simulink model "satellite"  (R2017a)
settings: Solver=FixedStepDiscrete  StartTime=0.0  StopTime=0.02  RelTol=1e-3
libraries: dspswit3 x9, commsynccomp2 x6, dspindex x3, commutil2 x3, dspmathops x3
(part 2 of 15)

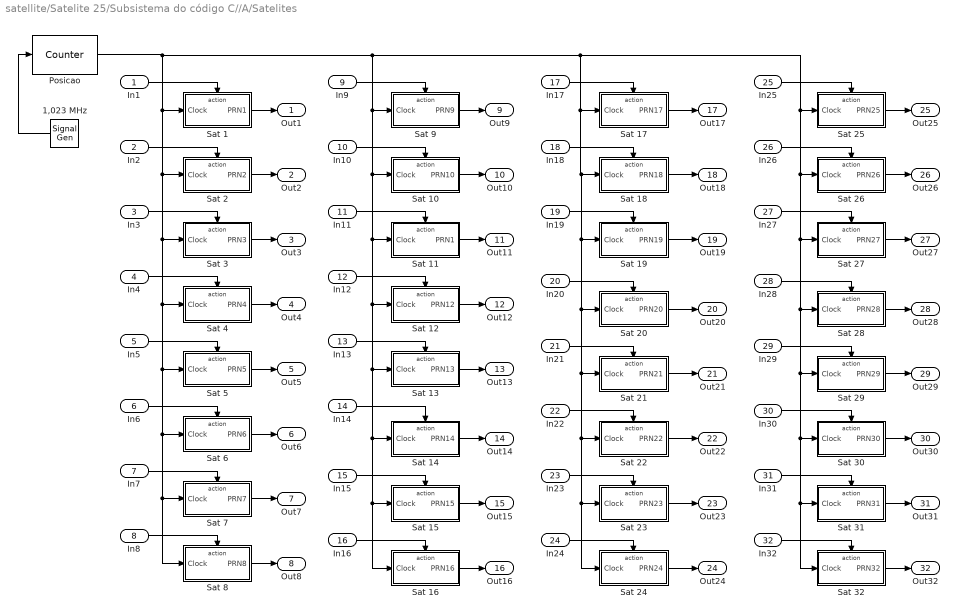
== system satellite/Satelite 25/Subsistema do código C//A/Satelites ==
  In1 : Inport
  In2 : Inport  Port=2
  In3 : Inport  Port=3
  In4 : Inport  Port=4
  In5 : Inport  Port=5
  In6 : Inport  Port=6
  In7 : Inport  Port=7
  In8 : Inport  Port=8
  In9 : Inport  Port=9
  In10 : Inport  Port=10
  In11 : Inport  Port=11
  In12 : Inport  Port=12
  In13 : Inport  Port=13
  In14 : Inport  Port=14
  In15 : Inport  Port=15
  In16 : Inport  Port=16
  In17 : Inport  Port=17
  In18 : Inport  Port=18
  In19 : Inport  Port=19
  In20 : Inport  Port=20
  In21 : Inport  Port=21
  In22 : Inport  Port=22
  In23 : Inport  Port=23
  In24 : Inport  Port=24
  In25 : Inport  Port=25
  In26 : Inport  Port=26
  In27 : Inport  Port=27
  In28 : Inport  Port=28
  In29 : Inport  Port=29
  In30 : Inport  Port=30
  In31 : Inport  Port=31
  In32 : Inport  Port=32
  1,023 MHz : SignalGenerator  WaveForm=square  Frequency=1.023e6
  Posicao : dspswit3/Counter  Direction=Up  CountEvent=Rising edge  CounterSize=User defined  MaxCount=1022  InitialCount=0  Output=Count  HitValue=32  ResetInput=off  SamplesPerFrame=1  Ts=1  CntDtype=double  HitDtype=Logical
  Sat 1 : Subsystem  TreatAsAtomicUnit=on
  Sat 10 : Subsystem  TreatAsAtomicUnit=on
  Sat 11 : Subsystem  TreatAsAtomicUnit=on
  Sat 12 : Subsystem  TreatAsAtomicUnit=on
  Sat 13 : Subsystem  TreatAsAtomicUnit=on
  Sat 14 : Subsystem  TreatAsAtomicUnit=on
  Sat 15 : Subsystem  TreatAsAtomicUnit=on
  Sat 16 : Subsystem  TreatAsAtomicUnit=on
  Sat 17 : Subsystem  TreatAsAtomicUnit=on
  Sat 18 : Subsystem  TreatAsAtomicUnit=on
  Sat 19 : Subsystem  TreatAsAtomicUnit=on
  Sat 2 : Subsystem  TreatAsAtomicUnit=on
  Sat 20 : Subsystem  TreatAsAtomicUnit=on
  Sat 21 : Subsystem  TreatAsAtomicUnit=on
  Sat 22 : Subsystem  TreatAsAtomicUnit=on
  Sat 23 : Subsystem  TreatAsAtomicUnit=on
  Sat 24 : Subsystem  TreatAsAtomicUnit=on
  Sat 25 : Subsystem  TreatAsAtomicUnit=on
  Sat 26 : Subsystem  TreatAsAtomicUnit=on
  Sat 27 : Subsystem  TreatAsAtomicUnit=on
  Sat 28 : Subsystem  TreatAsAtomicUnit=on
  Sat 29 : Subsystem  TreatAsAtomicUnit=on
  Sat 3 : Subsystem  TreatAsAtomicUnit=on
  Sat 30 : Subsystem  TreatAsAtomicUnit=on
  Sat 31 : Subsystem  TreatAsAtomicUnit=on
  Sat 32 : Subsystem  TreatAsAtomicUnit=on
  Sat 4 : Subsystem  TreatAsAtomicUnit=on
  Sat 5 : Subsystem  TreatAsAtomicUnit=on
  Sat 6 : Subsystem  TreatAsAtomicUnit=on
  Sat 7 : Subsystem  TreatAsAtomicUnit=on
  Sat 8 : Subsystem  TreatAsAtomicUnit=on
  Sat 9 : Subsystem  TreatAsAtomicUnit=on
  Out1 : Outport
  Out2 : Outport  Port=2
  Out3 : Outport  Port=3
  Out4 : Outport  Port=4
  Out5 : Outport  Port=5
  Out6 : Outport  Port=6
  Out7 : Outport  Port=7
  Out8 : Outport  Port=8
  Out9 : Outport  Port=9
  Out10 : Outport  Port=10
  Out11 : Outport  Port=11
  Out12 : Outport  Port=12
  Out13 : Outport  Port=13
  Out14 : Outport  Port=14
  Out15 : Outport  Port=15
  Out16 : Outport  Port=16
  Out17 : Outport  Port=17
  Out18 : Outport  Port=18
  Out19 : Outport  Port=19
  Out20 : Outport  Port=20
  Out21 : Outport  Port=21
  Out22 : Outport  Port=22
  Out23 : Outport  Port=23
  Out24 : Outport  Port=24
  Out25 : Outport  Port=25
  Out26 : Outport  Port=26
  Out27 : Outport  Port=27
  Out28 : Outport  Port=28
  Out29 : Outport  Port=29
  Out30 : Outport  Port=30
  Out31 : Outport  Port=31
  Out32 : Outport  Port=32
  wires:
  Sat 1/1(PRN1) -> Out1/1
  Sat 2/1(PRN2) -> Out2/1
  Sat 3/1(PRN3) -> Out3/1
  Sat 4/1(PRN4) -> Out4/1
  Sat 5/1(PRN5) -> Out5/1
  Sat 6/1(PRN6) -> Out6/1
  In1/1 -> Sat 1/Action
  In2/1 -> Sat 2/Action
  In3/1 -> Sat 3/Action
  In4/1 -> Sat 4/Action
  In5/1 -> Sat 5/Action
  In6/1 -> Sat 6/Action
  In8/1 -> Sat 8/Action
  In10/1 -> Sat 10/Action
  In7/1 -> Sat 7/Action
  Sat 8/1(PRN8) -> Out8/1
  Sat 11/1(PRN1) -> Out11/1
  Sat 10/1(PRN10) -> Out10/1
  In11/1 -> Sat 11/Action
  In9/1 -> Sat 9/Action
  Sat 12/1(PRN12) -> Out12/1
  Sat 9/1(PRN9) -> Out9/1
  Sat 7/1(PRN7) -> Out7/1
  In12/1 -> Sat 12/Action
  In14/1 -> Sat 14/Action
  In16/1 -> Sat 16/Action
  In13/1 -> Sat 13/Action
  Sat 14/1(PRN14) -> Out14/1
  Sat 17/1(PRN17) -> Out17/1
  Sat 16/1(PRN16) -> Out16/1
  In17/1 -> Sat 17/Action
  In15/1 -> Sat 15/Action
  Sat 18/1(PRN18) -> Out18/1
  Sat 15/1(PRN15) -> Out15/1
  Sat 13/1(PRN13) -> Out13/1
  In18/1 -> Sat 18/Action
  In20/1 -> Sat 20/Action
  In22/1 -> Sat 22/Action
  In19/1 -> Sat 19/Action
  Sat 20/1(PRN20) -> Out20/1
  Sat 23/1(PRN23) -> Out23/1
  Sat 22/1(PRN22) -> Out22/1
  In23/1 -> Sat 23/Action
  In21/1 -> Sat 21/Action
  Sat 24/1(PRN24) -> Out24/1
  Sat 21/1(PRN21) -> Out21/1
  Sat 19/1(PRN19) -> Out19/1
  In24/1 -> Sat 24/Action
  In26/1 -> Sat 26/Action
  In28/1 -> Sat 28/Action
  In25/1 -> Sat 25/Action
  Sat 26/1(PRN26) -> Out26/1
  Sat 29/1(PRN29) -> Out29/1
  Sat 28/1(PRN28) -> Out28/1
  In29/1 -> Sat 29/Action
  In27/1 -> Sat 27/Action
  Sat 30/1(PRN30) -> Out30/1
  Sat 27/1(PRN27) -> Out27/1
  Sat 25/1(PRN25) -> Out25/1
  In30/1 -> Sat 30/Action
  In32/1 -> Sat 32/Action
  Sat 32/1(PRN32) -> Out32/1
  Sat 31/1(PRN31) -> Out31/1
  In31/1 -> Sat 31/Action
  Posicao/1 -> Sat 8/1(Clock), Sat 7/1(Clock), Sat 6/1(Clock), Sat 5/1(Clock), Sat 4/1(Clock), Sat 3/1(Clock), Sat 2/1(Clock), Sat 1/1(Clock), Sat 25/1(Clock), Sat 26/1(Clock), Sat 28/1(Clock), Sat 29/1(Clock), Sat 30/1(Clock), Sat 31/1(Clock), Sat 32/1(Clock), Sat 27/1(Clock), Sat 24/1(Clock), Sat 23/1(Clock), Sat 22/1(Clock), Sat 21/1(Clock), Sat 20/1(Clock), Sat 19/1(Clock), Sat 18/1(Clock), Sat 17/1(Clock), Sat 9/1(Clock), Sat 10/1(Clock), Sat 16/1(Clock), Sat 15/1(Clock), Sat 14/1(Clock), Sat 13/1(Clock), Sat 12/1(Clock), Sat 11/1(Clock)
  1,023 MHz/1 -> Posicao/1

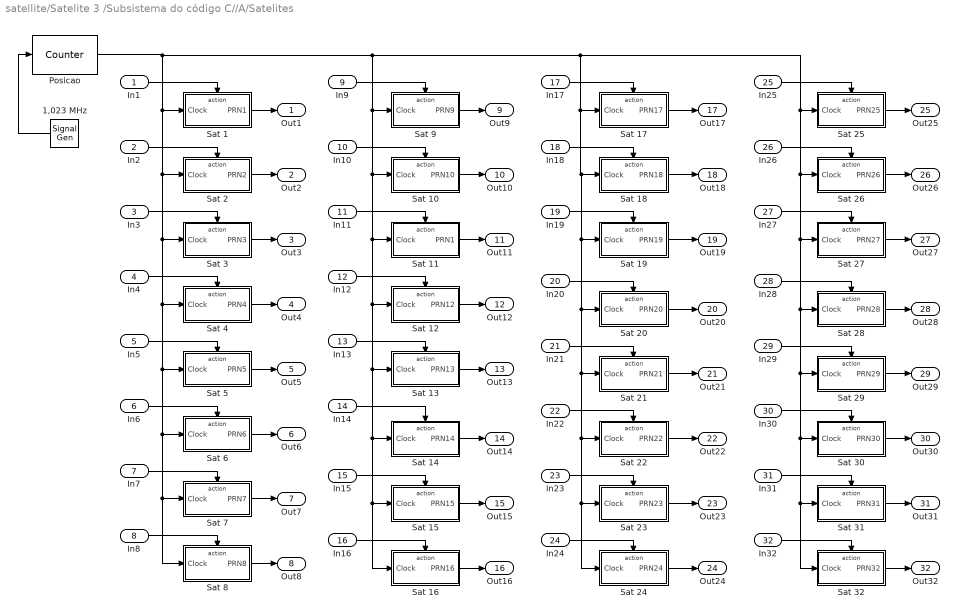
== system satellite/Satelite 3 /Subsistema do código C//A/Satelites ==
  In1 : Inport
  In2 : Inport  Port=2
  In3 : Inport  Port=3
  In4 : Inport  Port=4
  In5 : Inport  Port=5
  In6 : Inport  Port=6
  In7 : Inport  Port=7
  In8 : Inport  Port=8
  In9 : Inport  Port=9
  In10 : Inport  Port=10
  In11 : Inport  Port=11
  In12 : Inport  Port=12
  In13 : Inport  Port=13
  In14 : Inport  Port=14
  In15 : Inport  Port=15
  In16 : Inport  Port=16
  In17 : Inport  Port=17
  In18 : Inport  Port=18
  In19 : Inport  Port=19
  In20 : Inport  Port=20
  In21 : Inport  Port=21
  In22 : Inport  Port=22
  In23 : Inport  Port=23
  In24 : Inport  Port=24
  In25 : Inport  Port=25
  In26 : Inport  Port=26
  In27 : Inport  Port=27
  In28 : Inport  Port=28
  In29 : Inport  Port=29
  In30 : Inport  Port=30
  In31 : Inport  Port=31
  In32 : Inport  Port=32
  1,023 MHz : SignalGenerator  WaveForm=square  Frequency=1.023e6
  Posicao : dspswit3/Counter  Direction=Up  CountEvent=Rising edge  CounterSize=User defined  MaxCount=1022  InitialCount=0  Output=Count  HitValue=32  ResetInput=off  SamplesPerFrame=1  Ts=1  CntDtype=double  HitDtype=Logical
  Sat 1 : Subsystem  TreatAsAtomicUnit=on
  Sat 10 : Subsystem  TreatAsAtomicUnit=on
  Sat 11 : Subsystem  TreatAsAtomicUnit=on
  Sat 12 : Subsystem  TreatAsAtomicUnit=on
  Sat 13 : Subsystem  TreatAsAtomicUnit=on
  Sat 14 : Subsystem  TreatAsAtomicUnit=on
  Sat 15 : Subsystem  TreatAsAtomicUnit=on
  Sat 16 : Subsystem  TreatAsAtomicUnit=on
  Sat 17 : Subsystem  TreatAsAtomicUnit=on
  Sat 18 : Subsystem  TreatAsAtomicUnit=on
  Sat 19 : Subsystem  TreatAsAtomicUnit=on
  Sat 2 : Subsystem  TreatAsAtomicUnit=on
  Sat 20 : Subsystem  TreatAsAtomicUnit=on
  Sat 21 : Subsystem  TreatAsAtomicUnit=on
  Sat 22 : Subsystem  TreatAsAtomicUnit=on
  Sat 23 : Subsystem  TreatAsAtomicUnit=on
  Sat 24 : Subsystem  TreatAsAtomicUnit=on
  Sat 25 : Subsystem  TreatAsAtomicUnit=on
  Sat 26 : Subsystem  TreatAsAtomicUnit=on
  Sat 27 : Subsystem  TreatAsAtomicUnit=on
  Sat 28 : Subsystem  TreatAsAtomicUnit=on
  Sat 29 : Subsystem  TreatAsAtomicUnit=on
  Sat 3 : Subsystem  TreatAsAtomicUnit=on
  Sat 30 : Subsystem  TreatAsAtomicUnit=on
  Sat 31 : Subsystem  TreatAsAtomicUnit=on
  Sat 32 : Subsystem  TreatAsAtomicUnit=on
  Sat 4 : Subsystem  TreatAsAtomicUnit=on
  Sat 5 : Subsystem  TreatAsAtomicUnit=on
  Sat 6 : Subsystem  TreatAsAtomicUnit=on
  Sat 7 : Subsystem  TreatAsAtomicUnit=on
  Sat 8 : Subsystem  TreatAsAtomicUnit=on
  Sat 9 : Subsystem  TreatAsAtomicUnit=on
  Out1 : Outport
  Out2 : Outport  Port=2
  Out3 : Outport  Port=3
  Out4 : Outport  Port=4
  Out5 : Outport  Port=5
  Out6 : Outport  Port=6
  Out7 : Outport  Port=7
  Out8 : Outport  Port=8
  Out9 : Outport  Port=9
  Out10 : Outport  Port=10
  Out11 : Outport  Port=11
  Out12 : Outport  Port=12
  Out13 : Outport  Port=13
  Out14 : Outport  Port=14
  Out15 : Outport  Port=15
  Out16 : Outport  Port=16
  Out17 : Outport  Port=17
  Out18 : Outport  Port=18
  Out19 : Outport  Port=19
  Out20 : Outport  Port=20
  Out21 : Outport  Port=21
  Out22 : Outport  Port=22
  Out23 : Outport  Port=23
  Out24 : Outport  Port=24
  Out25 : Outport  Port=25
  Out26 : Outport  Port=26
  Out27 : Outport  Port=27
  Out28 : Outport  Port=28
  Out29 : Outport  Port=29
  Out30 : Outport  Port=30
  Out31 : Outport  Port=31
  Out32 : Outport  Port=32
  wires:
  Sat 1/1(PRN1) -> Out1/1
  Sat 2/1(PRN2) -> Out2/1
  Sat 3/1(PRN3) -> Out3/1
  Sat 4/1(PRN4) -> Out4/1
  Sat 5/1(PRN5) -> Out5/1
  Sat 6/1(PRN6) -> Out6/1
  In1/1 -> Sat 1/Action
  In2/1 -> Sat 2/Action
  In3/1 -> Sat 3/Action
  In4/1 -> Sat 4/Action
  In5/1 -> Sat 5/Action
  In6/1 -> Sat 6/Action
  In8/1 -> Sat 8/Action
  In10/1 -> Sat 10/Action
  In7/1 -> Sat 7/Action
  Sat 8/1(PRN8) -> Out8/1
  Sat 11/1(PRN1) -> Out11/1
  Sat 10/1(PRN10) -> Out10/1
  In11/1 -> Sat 11/Action
  In9/1 -> Sat 9/Action
  Sat 12/1(PRN12) -> Out12/1
  Sat 9/1(PRN9) -> Out9/1
  Sat 7/1(PRN7) -> Out7/1
  In12/1 -> Sat 12/Action
  In14/1 -> Sat 14/Action
  In16/1 -> Sat 16/Action
  In13/1 -> Sat 13/Action
  Sat 14/1(PRN14) -> Out14/1
  Sat 17/1(PRN17) -> Out17/1
  Sat 16/1(PRN16) -> Out16/1
  In17/1 -> Sat 17/Action
  In15/1 -> Sat 15/Action
  Sat 18/1(PRN18) -> Out18/1
  Sat 15/1(PRN15) -> Out15/1
  Sat 13/1(PRN13) -> Out13/1
  In18/1 -> Sat 18/Action
  In20/1 -> Sat 20/Action
  In22/1 -> Sat 22/Action
  In19/1 -> Sat 19/Action
  Sat 20/1(PRN20) -> Out20/1
  Sat 23/1(PRN23) -> Out23/1
  Sat 22/1(PRN22) -> Out22/1
  In23/1 -> Sat 23/Action
  In21/1 -> Sat 21/Action
  Sat 24/1(PRN24) -> Out24/1
  Sat 21/1(PRN21) -> Out21/1
  Sat 19/1(PRN19) -> Out19/1
  In24/1 -> Sat 24/Action
  In26/1 -> Sat 26/Action
  In28/1 -> Sat 28/Action
  In25/1 -> Sat 25/Action
  Sat 26/1(PRN26) -> Out26/1
  Sat 29/1(PRN29) -> Out29/1
  Sat 28/1(PRN28) -> Out28/1
  In29/1 -> Sat 29/Action
  In27/1 -> Sat 27/Action
  Sat 30/1(PRN30) -> Out30/1
  Sat 27/1(PRN27) -> Out27/1
  Sat 25/1(PRN25) -> Out25/1
  In30/1 -> Sat 30/Action
  In32/1 -> Sat 32/Action
  Sat 32/1(PRN32) -> Out32/1
  Sat 31/1(PRN31) -> Out31/1
  In31/1 -> Sat 31/Action
  Posicao/1 -> Sat 8/1(Clock), Sat 7/1(Clock), Sat 6/1(Clock), Sat 5/1(Clock), Sat 4/1(Clock), Sat 3/1(Clock), Sat 2/1(Clock), Sat 1/1(Clock), Sat 25/1(Clock), Sat 26/1(Clock), Sat 28/1(Clock), Sat 29/1(Clock), Sat 30/1(Clock), Sat 31/1(Clock), Sat 32/1(Clock), Sat 27/1(Clock), Sat 24/1(Clock), Sat 23/1(Clock), Sat 22/1(Clock), Sat 21/1(Clock), Sat 20/1(Clock), Sat 19/1(Clock), Sat 18/1(Clock), Sat 17/1(Clock), Sat 9/1(Clock), Sat 10/1(Clock), Sat 16/1(Clock), Sat 15/1(Clock), Sat 14/1(Clock), Sat 13/1(Clock), Sat 12/1(Clock), Sat 11/1(Clock)
  1,023 MHz/1 -> Posicao/1

== system satellite/Satelite 14 /Subsistema do código C//A/Satelites/Sat 1 ==
  Clock : Inport
  Action Port : ActionPort  ActionType=case
  Tabela de C/A : Lookup_n-D  NumberOfTableDimensions=1  BreakpointsForDimension1=[0,1,2,3,4,5,6,7,8,9,10,11,12,13,14,15,16,17,18,19,20,21,22,23,24,25,26,27,28,29,30,31,32,33,34,35,36,37,38,39,40,41,42,43,44,45,46,47,48,49,50,51,52,53,54,55,56,57,58,59,60,61,62,63,64,65,66,67,68,69,70,71,72,73,74,75,76,77,78,79,80,81,82,83,84,85,86,87,88,89,90,91,92,93,94,95,96,97,98,99,100,101,102,103,104,105,106,107,108,109,110,111,112,113,114,115,116,117,118,119,120,121,122,123,124,125,126,127,128,129,130,131,132,133,134,135,136,137,138,139,140,141,142,143,144,145,146,147,148,149,150,151,152,153,154,155,156,157,158,159,160,161,162,163,164,165,166,167,168,169,170,171,172,173,174,175,176,177,178,179,180,181,182,183,184,185,186,187,188,189,190,191,192,193,194,195,196,197,198,199,200,201,202,203,204,205,206,207,208,209,210,211,212,213,214,215,216,217,218,219,220,221,222,223,224,225,226,227,228,229,230,231,232,233,234,235,236,237,238,239,240,241,242,243,244,245,246,247,248,249,250,251,252,253,254,255,256,257,258,259,260,261,262,263,264,265,266,267,268,269,270,271,272,273,274,275,276,277,278,279,280,281,282,283,284,285,286,287,288,289,290,291,292,293,294,295,296,297,298,299,300,301,302,303,304,305,306,307,308,309,310,311,312,313,314,315,316,317,318,319,320,321,322,323,324,325,326,327,328,329,330,331,332,333,334,335,336,337,338,339,340,341,342,343,344,345,346,347,348,349,350,351,352,353,354,355,356,357,358,359,360,361,362,363,364,365,366,367,368,369,370,371,372,373,374,375,376,377,378,379,380,381,382,383,384,385,386,387,388,389,390,391,392,393,394,395,396,397,398,399,400,401,402,403,404,405,406,407,408,409,410,411,412,413,414,415,416,417,418,419,420,421,422,423,424,425,426,427,428,429,430,431,432,433,434,435,436,437,438,439,440,441,442,443,444,445,446,447,448,449,450,451,452,453,454,455,456,457,458,459,460,461,462,463,464,465,466,467,468,469,470,471,472,473,474,475,476,477,478,479,480,481,482,483,484,485,486,487,488,489,490,491,492,493,494,495,496,497,498,499,500,501,502,503,504,505,506,507,508,509,510,511,512,513,514,515,516,517,518,519,520,521,522,523,524,525,526,527,528,529,530,531,532,533,534,535,536,537,538,539,540,541,542,543,544,545,546,547,548,549,550,551,552,553,554,555,556,557,558,559,560,561,562,563,564,565,566,567,568,569,570,571,572,573,574,575,576,577,578,579,580,581,582,583,584,585,586,587,588,589,590,591,592,593,594,595,596,597,598,599,600,601,602,603,604,605,606,607,608,609,610,611,612,613,614,615,616,617,618,619,620,621,622,623,624,625,626,627,628,629,630,631,632,633,634,635,636,637,638,639,640,641,642,643,644,645,646,647,648,649,650,651,652,653,654,655,656,657,658,659,660,661,662,663,664,665,666,667,668,669,670,671,672,673,674,675,676,677,678,679,680,681,682,683,684,685,686,687,688,689,690,691,692,693,694,695,696,697,698,699,700,701,702,703,704,705,706,707,708,709,710,711,712,713,714,715,716,717,718,719,720,721,722,723,724,725,726,727,728,729,730,731,732,733,734,735,736,737,738,739,740,741,742,743,744,745,746,747,748,749,750,751,752,753,754,755,756,757,758,759,760,761,762,763,764,765,766,767,768,769,770,771,772,773,774,775,776,777,778,779,780,781,782,783,784,785,786,787,788,789,790,791,792,793,794,795,796,797,798,799,800,801,802,803,804,805,806,807,808,809,810,811,812,813,814,815,816,817,818,819,820,821,822,823,824,825,826,827,828,829,830,831,832,833,834,835,836,837,838,839,840,841,842,843,844,845,846,847,848,849,850,851,852,853,854,855,856,857,858,859,860,861,862,863,864,865,866,867,868,869,870,871,872,873,874,875,876,877,878,879,880,881,882,883,884,885,886,887,888,889,890,891,892,893,894,895,896,897,898,899,900,901,902,903,904,905,906,907,908,909,910,911,912,913,914,915,916,917,918,919,920,921,922,923,924,925,926,927,928,929,930,931,932,933,934,935,936,937,938,939,940,941,942,943,944,945,946,947,948,949,950,951,952,953,954,955,956,957,958,959,960,961,962,963,964,965,966,967,968,969,970,971,972,973,974,975,976,977,978,979,980,981,982,983,984,985,986,987,988,989,990,991,992,993,994,995,996,997,998,999,1000,1001,1002,1003,1004,1005,1006,1007,1008,1009,1010,1011,1012,1013,1014,1015,1016,1017,1018,1019,1020,1021,1022]  Table=[1,1,-1,-1,1,-1,-1,-1,-1,-1,1,1,1,-1,-1,1,-1,1,-1,-1,1,-1,-1,1,1,1,1,-1,-1,1,-1,1,-1,-1,-1,1,-1,-1,1,1,1,1,1,-1,1,-1,1,-1,1,1,-1,1,-1,-1,-1,1,-1,-1,-1,1,-1,1,-1,1,-1,1,-1,1,1,-1,-1,1,-1,-1,-1,1,1,1,1,-1,1,-1,-1,1,1,1,1,1,1,-1,1,1,-1,1,1,1,-1,-1,1,1,-1,1,1,1,1,1,-1,-1,1,-1,1,-1,1,-1,1,-1,-1,-1,-1,1,-1,-1,-1,-1,-1,-1,-1,-1,1,1,1,-1,1,-1,1,-1,-1,1,-1,-1,-1,1,-1,-1,1,1,-1,1,1,1,1,-1,-1,-1,-1,-1,1,1,1,1,-1,1,-1,1,1,1,-1,-1,1,1,-1,-1,1,1,1,1,-1,1,1,-1,-1,-1,-1,-1,-1,-1,1,-1,1,1,1,1,-1,-1,1,1,1,1,1,-1,1,-1,1,-1,-1,1,1,-1,-1,-1,1,-1,1,1,-1,1,1,1,-1,-1,-1,1,1,-1,1,1,1,1,-1,1,-1,1,-1,-1,-1,1,-1,1,-1,1,1,-1,-1,-1,-1,-1,1,-1,-1,-1,-1,-1,-1,-1,-1,1,-1,-1,-1,-1,-1,-1,1,1,-1,-1,-1,1,1,1,-1,1,1,-1,-1,-1,-1,-1,-1,1,1,1,-1,-1,-1,1,1,-1,1,1,1,1,1,1,1,1,1,-1,1,-1,-1,1,1,1,-1,1,-1,-1,1,-1,1,1,-1,1,1,-1,-1,-1,-1,1,-1,1,-1,1,-1,1,1,-1,-1,-1,1,-1,-1,1,1,1,-1,-1,1,-1,1,1,-1,1,1,1,-1,1,1,-1,-1,-1,1,1,1,-1,1,1,1,-1,1,1,1,1,-1,-1,-1,-1,1,1,-1,1,1,-1,-1,-1,-1,1,1,-1,-1,1,-1,-1,1,-1,-1,1,-1,-1,-1,-1,-1,1,1,-1,1,1,-1,1,-1,-1,1,-1,1,1,-1,1,1,1,1,-1,-1,-1,1,-1,1,1,1,-1,-1,-1,-1,-1,-1,1,-1,1,-1,-1,1,-1,-1,1,1,1,1,1,1,-1,-1,-1,-1,-1,1,-1,1,-1,1,-1,1,1,1,-1,-1,1,1,1,1,1,-1,1,-1,1,1,1,1,1,-1,-1,1,1,-1,-1,1,1,-1,-1,-1,1,1,1,-1,-1,-1,1,1,-1,1,1,-1,1,-1,1,-1,1,-1,1,1,-1,1,1,-1,-1,-1,1,1,-1,1,1,1,-1,1,1,1,-1,-1,-1,-1,-1,-1,-1,-1,-1,-1,-1,1,-1,1,1,-1,-1,1,1,-1,1,1,-1,-1,1,1,1,-1,1,1,-1,1,-1,-1,-1,-1,-1,1,-1,1,-1,1,-1,1,1,1,-1,1,-1,1,1,1,-1,1,-1,-1,1,-1,1,-1,-1,-1,1,1,1,-1,-1,1,1,1,-1,-1,-1,1,-1,-1,1,-1,1,-1,-1,-1,1,-1,1,-1,-1,1,-1,1,1,-1,1,-1,-1,-1,-1,1,-1,1,-1,1,1,-1,1,1,-1,1,-1,1,1,-1,1,1,-1,-1,-1,1,1,1,-1,-1,1,1,1,1,-1,1,1,-1,-1,1,-1,-1,-1,-1,1,1,1,1,1,1,-1,-1,1,-1,1,1,-1,1,-1,-1,-1,1,-1,-1,-1,-1,1,1,1,1,1,-1,1,-1,1,-1,1,1,1,-1,-1,1,1,-1,-1,1,-1,-1,1,-1,-1,1,-1,-1,1,-1,1,1,1,1,1,1,1,1,1,1,-1,-1,-1,-1,1,1,1,1,1,-1,1,1,1,1,-1,-1,-1,1,1,-1,1,1,1,-1,-1,1,-1,1,1,-1,-1,-1,-1,1,1,1,-1,-1,1,-1,1,-1,1,-1,-1,-1,-1,1,-1,1,-1,-1,1,-1,1,-1,1,1,1,1,1,1,-1,-1,-1,1,1,1,1,-1,1,1,-1,1,-1,-1,1,1,1,-1,1,1,-1,-1,1,1,1,1,1,1,-1,1,1,1,1,1,-1,1,-1,-1,-1,1,1,-1,-1,-1,1,1,1,1,1,-1,-1,-1,-1,-1,-1,-1,1,-1,-1,1,-1,1,-1,-1,-1,1,-1,1,1,-1,1,-1,-1,-1,1,-1,-1,-1,1,-1,-1,1,1,-1,1,1,-1,-1,-1,-1,-1,-1,1,1,1,-1,1,1,-1,1,-1,-1,-1,1,1,-1,1,-1,-1,-1,1,-1,-1,1,-1,-1,-1,1,1,1,-1,-1,-1,1,-1,1,1,-1,-1,1,1,-1,-1,1,-1,-1,1,1,1,1,-1,-1,1,1,-1,1,1,1,1,1,1,-1,-1,1,1,-1,-1,1,-1,1,-1,-1,1,1,-1,1,-1,-1,1,1,-1,1,-1,1,1,1,1,-1,-1,1,1,-1,1,1,-1,1,-1,1,-1,-1,1,1,1,-1,1,1,1,1,-1,-1,-1,1,1,-1,1,-1,1,-1,-1,-1,1,-1,-1,-1,-1,1,-1,-1,-1,1,-1,-1,1,-1,-1,1,1,1,-1,-1,-1,-1,1,1,1,-1,-1,1,-1,1,-1,-1,-1,1,-1,-1,-1,-1]  InternalRulePriority=Speed  RndMeth=Simplest  InputSameDT=on
  PRN1 : Outport
  wires:
  Clock/1 -> Tabela de C/A/1
  Tabela de C/A/1 -> PRN1/1

== system satellite/Satelite 14 /Subsistema do código C//A/Satelites/Sat 10 ==
  Clock : Inport
  Action Port : ActionPort  ActionType=case
  Tabela de C/A : Lookup_n-D  NumberOfTableDimensions=1  BreakpointsForDimension1=[0,1,2,3,4,5,6,7,8,9,10,11,12,13,14,15,16,17,18,19,20,21,22,23,24,25,26,27,28,29,30,31,32,33,34,35,36,37,38,39,40,41,42,43,44,45,46,47,48,49,50,51,52,53,54,55,56,57,58,59,60,61,62,63,64,65,66,67,68,69,70,71,72,73,74,75,76,77,78,79,80,81,82,83,84,85,86,87,88,89,90,91,92,93,94,95,96,97,98,99,100,101,102,103,104,105,106,107,108,109,110,111,112,113,114,115,116,117,118,119,120,121,122,123,124,125,126,127,128,129,130,131,132,133,134,135,136,137,138,139,140,141,142,143,144,145,146,147,148,149,150,151,152,153,154,155,156,157,158,159,160,161,162,163,164,165,166,167,168,169,170,171,172,173,174,175,176,177,178,179,180,181,182,183,184,185,186,187,188,189,190,191,192,193,194,195,196,197,198,199,200,201,202,203,204,205,206,207,208,209,210,211,212,213,214,215,216,217,218,219,220,221,222,223,224,225,226,227,228,229,230,231,232,233,234,235,236,237,238,239,240,241,242,243,244,245,246,247,248,249,250,251,252,253,254,255,256,257,258,259,260,261,262,263,264,265,266,267,268,269,270,271,272,273,274,275,276,277,278,279,280,281,282,283,284,285,286,287,288,289,290,291,292,293,294,295,296,297,298,299,300,301,302,303,304,305,306,307,308,309,310,311,312,313,314,315,316,317,318,319,320,321,322,323,324,325,326,327,328,329,330,331,332,333,334,335,336,337,338,339,340,341,342,343,344,345,346,347,348,349,350,351,352,353,354,355,356,357,358,359,360,361,362,363,364,365,366,367,368,369,370,371,372,373,374,375,376,377,378,379,380,381,382,383,384,385,386,387,388,389,390,391,392,393,394,395,396,397,398,399,400,401,402,403,404,405,406,407,408,409,410,411,412,413,414,415,416,417,418,419,420,421,422,423,424,425,426,427,428,429,430,431,432,433,434,435,436,437,438,439,440,441,442,443,444,445,446,447,448,449,450,451,452,453,454,455,456,457,458,459,460,461,462,463,464,465,466,467,468,469,470,471,472,473,474,475,476,477,478,479,480,481,482,483,484,485,486,487,488,489,490,491,492,493,494,495,496,497,498,499,500,501,502,503,504,505,506,507,508,509,510,511,512,513,514,515,516,517,518,519,520,521,522,523,524,525,526,527,528,529,530,531,532,533,534,535,536,537,538,539,540,541,542,543,544,545,546,547,548,549,550,551,552,553,554,555,556,557,558,559,560,561,562,563,564,565,566,567,568,569,570,571,572,573,574,575,576,577,578,579,580,581,582,583,584,585,586,587,588,589,590,591,592,593,594,595,596,597,598,599,600,601,602,603,604,605,606,607,608,609,610,611,612,613,614,615,616,617,618,619,620,621,622,623,624,625,626,627,628,629,630,631,632,633,634,635,636,637,638,639,640,641,642,643,644,645,646,647,648,649,650,651,652,653,654,655,656,657,658,659,660,661,662,663,664,665,666,667,668,669,670,671,672,673,674,675,676,677,678,679,680,681,682,683,684,685,686,687,688,689,690,691,692,693,694,695,696,697,698,699,700,701,702,703,704,705,706,707,708,709,710,711,712,713,714,715,716,717,718,719,720,721,722,723,724,725,726,727,728,729,730,731,732,733,734,735,736,737,738,739,740,741,742,743,744,745,746,747,748,749,750,751,752,753,754,755,756,757,758,759,760,761,762,763,764,765,766,767,768,769,770,771,772,773,774,775,776,777,778,779,780,781,782,783,784,785,786,787,788,789,790,791,792,793,794,795,796,797,798,799,800,801,802,803,804,805,806,807,808,809,810,811,812,813,814,815,816,817,818,819,820,821,822,823,824,825,826,827,828,829,830,831,832,833,834,835,836,837,838,839,840,841,842,843,844,845,846,847,848,849,850,851,852,853,854,855,856,857,858,859,860,861,862,863,864,865,866,867,868,869,870,871,872,873,874,875,876,877,878,879,880,881,882,883,884,885,886,887,888,889,890,891,892,893,894,895,896,897,898,899,900,901,902,903,904,905,906,907,908,909,910,911,912,913,914,915,916,917,918,919,920,921,922,923,924,925,926,927,928,929,930,931,932,933,934,935,936,937,938,939,940,941,942,943,944,945,946,947,948,949,950,951,952,953,954,955,956,957,958,959,960,961,962,963,964,965,966,967,968,969,970,971,972,973,974,975,976,977,978,979,980,981,982,983,984,985,986,987,988,989,990,991,992,993,994,995,996,997,998,999,1000,1001,1002,1003,1004,1005,1006,1007,1008,1009,1010,1011,1012,1013,1014,1015,1016,1017,1018,1019,1020,1021,1022]  Table=[1,1,-1,1,-1,-1,-1,1,-1,-1,1,-1,1,-1,-1,-1,1,-1,-1,1,1,1,-1,-1,-1,-1,1,1,-1,1,1,-1,1,-1,-1,-1,-1,1,-1,-1,-1,-1,-1,-1,1,-1,-1,-1,-1,1,-1,-1,-1,1,1,1,-1,1,1,-1,-1,1,1,-1,1,1,-1,1,-1,-1,1,-1,-1,-1,1,1,-1,-1,-1,-1,-1,-1,1,-1,1,1,-1,1,1,1,1,-1,-1,1,1,1,1,-1,1,-1,1,1,-1,-1,1,1,1,1,1,1,-1,1,-1,-1,-1,-1,-1,-1,1,-1,1,-1,-1,-1,-1,1,-1,1,1,-1,1,-1,-1,-1,1,-1,1,1,1,-1,-1,1,-1,-1,1,-1,-1,1,1,1,1,1,-1,-1,-1,1,1,1,-1,-1,-1,1,1,-1,-1,1,1,1,1,1,1,-1,-1,1,-1,-1,-1,-1,-1,-1,1,1,1,1,1,-1,-1,-1,1,1,1,-1,-1,1,-1,1,-1,1,-1,1,-1,-1,-1,1,-1,1,1,-1,-1,1,1,1,-1,1,-1,1,1,1,-1,-1,-1,1,-1,-1,-1,-1,-1,1,1,-1,1,1,1,1,1,-1,1,1,-1,1,-1,1,1,1,1,-1,1,-1,-1,1,-1,-1,-1,-1,1,-1,1,1,1,1,1,1,1,-1,1,1,-1,1,1,1,1,-1,-1,1,-1,1,-1,-1,1,-1,1,1,1,-1,1,-1,1,-1,1,-1,1,-1,-1,-1,1,1,-1,-1,-1,-1,1,1,1,1,-1,-1,1,-1,1,-1,-1,-1,-1,-1,-1,1,-1,1,-1,1,-1,-1,-1,-1,1,-1,-1,-1,-1,1,1,-1,-1,-1,-1,1,1,-1,1,1,-1,1,1,-1,-1,1,-1,1,-1,1,-1,-1,1,1,1,1,-1,-1,1,1,-1,1,-1,-1,1,-1,1,1,1,-1,-1,-1,-1,-1,-1,-1,-1,-1,1,1,1,-1,1,1,1,-1,1,-1,-1,-1,-1,1,1,-1,-1,-1,1,-1,1,-1,1,1,-1,1,1,1,-1,1,1,1,-1,1,1,1,1,-1,1,-1,1,-1,-1,1,-1,1,1,1,1,-1,1,-1,1,1,1,1,-1,-1,1,-1,-1,-1,1,-1,1,-1,1,1,-1,1,-1,1,1,1,-1,-1,-1,-1,-1,1,-1,1,-1,-1,-1,1,1,1,1,1,1,1,1,-1,1,1,-1,-1,1,1,1,-1,-1,1,-1,1,-1,-1,-1,-1,-1,1,-1,-1,-1,-1,-1,-1,1,-1,-1,-1,-1,1,1,-1,-1,1,1,-1,-1,-1,-1,1,-1,1,-1,-1,1,-1,1,-1,1,1,-1,1,-1,-1,1,-1,1,-1,-1,1,1,1,1,-1,-1,-1,1,-1,-1,1,-1,-1,1,-1,1,-1,1,1,-1,1,1,-1,1,1,-1,-1,1,-1,-1,1,-1,1,1,-1,-1,1,-1,-1,1,-1,-1,-1,-1,-1,1,-1,-1,-1,-1,-1,-1,1,-1,-1,-1,-1,-1,1,1,-1,-1,-1,1,-1,-1,1,1,1,-1,1,1,1,-1,-1,1,1,1,1,1,1,-1,1,1,1,1,1,1,1,1,1,1,1,-1,1,1,-1,1,-1,1,-1,1,1,1,-1,1,-1,1,-1,1,1,1,1,-1,1,1,-1,-1,-1,1,1,-1,1,1,1,-1,-1,1,1,1,1,-1,1,-1,1,1,1,-1,-1,1,-1,1,-1,-1,-1,1,1,-1,1,1,-1,-1,-1,-1,1,1,-1,1,1,1,-1,1,1,-1,1,1,-1,1,1,1,1,-1,1,-1,1,-1,1,-1,-1,-1,1,1,-1,1,-1,-1,-1,-1,-1,1,1,-1,1,1,1,1,1,-1,-1,-1,1,1,1,-1,1,1,-1,-1,-1,1,1,1,1,-1,1,-1,1,1,-1,1,-1,-1,1,1,1,1,-1,-1,1,-1,-1,1,-1,-1,1,-1,-1,-1,-1,1,-1,-1,1,1,1,1,-1,1,-1,1,1,1,-1,-1,1,-1,1,-1,1,-1,-1,1,1,-1,-1,-1,-1,1,-1,-1,-1,1,-1,1,1,1,-1,1,-1,-1,1,1,1,1,-1,1,1,-1,-1,1,-1,1,1,1,-1,1,-1,-1,1,-1,1,1,1,-1,-1,-1,-1,1,1,-1,-1,1,-1,1,-1,1,-1,1,1,1,1,-1,-1,1,1,-1,1,-1,1,-1,1,-1,1,-1,1,1,1,-1,1,1,1,-1,1,1,-1,-1,1,-1,-1,-1,1,1,-1,-1,-1,-1,-1,1,1,1,1,-1,-1,-1,-1,1,1,1,-1,-1,-1,1,1,1,1,-1,-1,1,1,1,1,1,1,1,1,1,1,1,1,-1,1,-1,1,-1,1,1,-1,1,-1,1,-1,-1,-1,-1,1,1,-1,-1,-1,-1,1,-1,-1,-1,-1,1,-1,1,-1,-1,-1,-1,-1,1,-1,1,-1,1,1,-1,1,-1,-1,-1,-1,-1,1,1,1,1,1,1,1,1,1,1,-1,-1,1,-1,1,-1,-1,-1,1,1,1,1,-1,1,1,1,-1,1,1,1,1,-1,-1,1,-1,1,-1,1,-1,-1,1,1,-1,-1,-1,1,1,-1,-1,-1,-1,-1,-1,-1,-1,-1]  InternalRulePriority=Speed  RndMeth=Simplest  InputSameDT=on
  PRN10 : Outport
  wires:
  Clock/1 -> Tabela de C/A/1
  Tabela de C/A/1 -> PRN10/1

== system satellite/Satelite 14 /Subsistema do código C//A/Satelites/Sat 11 ==
  Clock : Inport
  Action Port : ActionPort  ActionType=case
  Tabela de C/A : Lookup_n-D  NumberOfTableDimensions=1  BreakpointsForDimension1=[0,1,2,3,4,5,6,7,8,9,10,11,12,13,14,15,16,17,18,19,20,21,22,23,24,25,26,27,28,29,30,31,32,33,34,35,36,37,38,39,40,41,42,43,44,45,46,47,48,49,50,51,52,53,54,55,56,57,58,59,60,61,62,63,64,65,66,67,68,69,70,71,72,73,74,75,76,77,78,79,80,81,82,83,84,85,86,87,88,89,90,91,92,93,94,95,96,97,98,99,100,101,102,103,104,105,106,107,108,109,110,111,112,113,114,115,116,117,118,119,120,121,122,123,124,125,126,127,128,129,130,131,132,133,134,135,136,137,138,139,140,141,142,143,144,145,146,147,148,149,150,151,152,153,154,155,156,157,158,159,160,161,162,163,164,165,166,167,168,169,170,171,172,173,174,175,176,177,178,179,180,181,182,183,184,185,186,187,188,189,190,191,192,193,194,195,196,197,198,199,200,201,202,203,204,205,206,207,208,209,210,211,212,213,214,215,216,217,218,219,220,221,222,223,224,225,226,227,228,229,230,231,232,233,234,235,236,237,238,239,240,241,242,243,244,245,246,247,248,249,250,251,252,253,254,255,256,257,258,259,260,261,262,263,264,265,266,267,268,269,270,271,272,273,274,275,276,277,278,279,280,281,282,283,284,285,286,287,288,289,290,291,292,293,294,295,296,297,298,299,300,301,302,303,304,305,306,307,308,309,310,311,312,313,314,315,316,317,318,319,320,321,322,323,324,325,326,327,328,329,330,331,332,333,334,335,336,337,338,339,340,341,342,343,344,345,346,347,348,349,350,351,352,353,354,355,356,357,358,359,360,361,362,363,364,365,366,367,368,369,370,371,372,373,374,375,376,377,378,379,380,381,382,383,384,385,386,387,388,389,390,391,392,393,394,395,396,397,398,399,400,401,402,403,404,405,406,407,408,409,410,411,412,413,414,415,416,417,418,419,420,421,422,423,424,425,426,427,428,429,430,431,432,433,434,435,436,437,438,439,440,441,442,443,444,445,446,447,448,449,450,451,452,453,454,455,456,457,458,459,460,461,462,463,464,465,466,467,468,469,470,471,472,473,474,475,476,477,478,479,480,481,482,483,484,485,486,487,488,489,490,491,492,493,494,495,496,497,498,499,500,501,502,503,504,505,506,507,508,509,510,511,512,513,514,515,516,517,518,519,520,521,522,523,524,525,526,527,528,529,530,531,532,533,534,535,536,537,538,539,540,541,542,543,544,545,546,547,548,549,550,551,552,553,554,555,556,557,558,559,560,561,562,563,564,565,566,567,568,569,570,571,572,573,574,575,576,577,578,579,580,581,582,583,584,585,586,587,588,589,590,591,592,593,594,595,596,597,598,599,600,601,602,603,604,605,606,607,608,609,610,611,612,613,614,615,616,617,618,619,620,621,622,623,624,625,626,627,628,629,630,631,632,633,634,635,636,637,638,639,640,641,642,643,644,645,646,647,648,649,650,651,652,653,654,655,656,657,658,659,660,661,662,663,664,665,666,667,668,669,670,671,672,673,674,675,676,677,678,679,680,681,682,683,684,685,686,687,688,689,690,691,692,693,694,695,696,697,698,699,700,701,702,703,704,705,706,707,708,709,710,711,712,713,714,715,716,717,718,719,720,721,722,723,724,725,726,727,728,729,730,731,732,733,734,735,736,737,738,739,740,741,742,743,744,745,746,747,748,749,750,751,752,753,754,755,756,757,758,759,760,761,762,763,764,765,766,767,768,769,770,771,772,773,774,775,776,777,778,779,780,781,782,783,784,785,786,787,788,789,790,791,792,793,794,795,796,797,798,799,800,801,802,803,804,805,806,807,808,809,810,811,812,813,814,815,816,817,818,819,820,821,822,823,824,825,826,827,828,829,830,831,832,833,834,835,836,837,838,839,840,841,842,843,844,845,846,847,848,849,850,851,852,853,854,855,856,857,858,859,860,861,862,863,864,865,866,867,868,869,870,871,872,873,874,875,876,877,878,879,880,881,882,883,884,885,886,887,888,889,890,891,892,893,894,895,896,897,898,899,900,901,902,903,904,905,906,907,908,909,910,911,912,913,914,915,916,917,918,919,920,921,922,923,924,925,926,927,928,929,930,931,932,933,934,935,936,937,938,939,940,941,942,943,944,945,946,947,948,949,950,951,952,953,954,955,956,957,958,959,960,961,962,963,964,965,966,967,968,969,970,971,972,973,974,975,976,977,978,979,980,981,982,983,984,985,986,987,988,989,990,991,992,993,994,995,996,997,998,999,1000,1001,1002,1003,1004,1005,1006,1007,1008,1009,1010,1011,1012,1013,1014,1015,1016,1017,1018,1019,1020,1021,1022]  Table=[1 1 1 -1 1 -1 -1 -1 1 -1 1 1 -1 -1 -1 -1 1 1 -1 1 -1 1 -1 -1 -1 1 1 1 -1 -1 -1 -1 1 -1 1 -1 -1 1 -1 -1 -1 -1 1 1 1 -1 1 -1 -1 1 1 -1 -1 1 -1 -1 1 1 -1 -1 1 1 -1 1 -1 1 1 1 -1 1 -1 1 -1 -1 -1 1 1 1 1 1 1 1 1 -1 1 -1 -1 -1 1 1 -1 -1 1 -1 1 1 -1 1 -1 -1 1 -1 1 1 1 1 1 -1 1 -1 1 1 -1 1 -1 1 1 1 1 1 1 1 1 -1 -1 -1 -1 1 -1 -1 -1 -1 -1 -1 1 1 1 1 -1 1 -1 -1 1 -1 1 1 1 1 -1 -1 -1 -1 -1 1 -1 1 1 -1 1 1 -1 1 1 -1 1 1 -1 1 -1 1 1 1 -1 1 -1 1 -1 1 -1 -1 1 1 1 1 -1 -1 -1 -1 1 1 -1 -1 -1 1 1 1 -1 -1 1 1 -1 1 1 -1 -1 -1 -1 -1 -1 -1 1 -1 -1 -1 1 1 -1 -1 -1 1 1 -1 1 1 -1 1 -1 1 1 -1 -1 1 -1 -1 1 1 1 -1 1 -1 -1 -1 -1 1 1 -1 1 -1 1 1 1 1 -1 -1 1 -1 1 1 1 1 1 -1 1 1 -1 -1 -1 -1 -1 -1 1 1 1 -1 1 -1 -1 -1 1 1 -1 -1 -1 1 1 -1 1 -1 -1 -1 1 -1 -1 1 -1 -1 1 1 1 1 -1 1 -1 -1 1 -1 1 -1 1 1 1 1 1 -1 1 1 -1 -1 1 1 -1 1 -1 1 -1 -1 -1 -1 1 1 -1 1 1 -1 -1 -1 1 1 1 -1 -1 1 1 -1 1 -1 -1 1 -1 -1 1 -1 -1 -1 -1 1 1 -1 1 1 1 1 1 1 -1 1 1 1 -1 -1 -1 -1 1 1 -1 1 -1 -1 -1 -1 1 1 -1 -1 1 -1 1 1 1 -1 -1 1 1 -1 1 1 -1 -1 -1 1 1 -1 1 -1 1 -1 1 1 -1 1 1 -1 1 1 1 -1 -1 -1 -1 1 1 -1 1 1 1 -1 -1 -1 1 -1 -1 -1 -1 -1 -1 -1 -1 1 1 1 -1 1 -1 -1 1 1 -1 1 -1 -1 -1 -1 1 -1 -1 -1 1 1 -1 1 1 -1 1 -1 1 -1 -1 -1 1 1 -1 1 1 -1 1 -1 -1 -1 1 1 -1 -1 -1 1 1 1 1 1 1 1 -1 1 -1 -1 1 1 1 1 -1 -1 1 1 1 -1 -1 1 1 1 1 -1 1 -1 1 -1 1 1 -1 1 -1 1 1 1 1 1 1 1 1 1 1 -1 1 1 -1 1 -1 1 1 1 1 1 -1 -1 -1 -1 1 -1 1 1 -1 -1 1 -1 1 1 1 -1 -1 1 1 1 1 1 1 1 1 -1 -1 1 1 -1 -1 -1 -1 1 1 1 1 1 1 1 -1 -1 1 1 -1 -1 -1 1 1 1 -1 -1 -1 -1 -1 1 -1 1 -1 -1 1 -1 -1 1 1 1 -1 -1 1 -1 -1 1 1 1 1 -1 -1 -1 -1 1 1 -1 1 -1 -1 1 1 1 -1 1 -1 -1 -1 -1 1 -1 1 1 1 -1 -1 1 -1 -1 1 -1 1 1 1 1 -1 -1 1 1 -1 1 -1 1 1 1 -1 1 1 -1 -1 -1 -1 1 -1 1 1 -1 1 -1 -1 1 -1 1 1 1 -1 -1 -1 -1 1 1 1 -1 1 -1 1 1 1 1 -1 -1 1 1 1 -1 1 -1 1 -1 1 -1 1 -1 -1 1 -1 -1 -1 1 -1 -1 -1 -1 -1 1 -1 1 1 -1 1 -1 1 1 -1 1 -1 1 -1 1 -1 -1 1 -1 1 1 1 1 1 -1 -1 -1 -1 -1 -1 1 1 -1 -1 -1 1 1 -1 1 1 1 -1 -1 1 -1 -1 1 1 -1 -1 1 1 1 -1 -1 1 -1 1 1 1 -1 1 -1 -1 -1 1 -1 -1 1 -1 -1 1 -1 1 -1 -1 1 -1 -1 -1 1 -1 -1 1 -1 1 1 -1 -1 -1 -1 1 -1 1 1 -1 1 1 1 1 -1 1 1 -1 -1 -1 1 -1 -1 -1 -1 1 -1 1 -1 -1 -1 1 -1 -1 -1 1 -1 1 -1 1 -1 -1 -1 1 -1 -1 -1 1 -1 -1 -1 1 1 1 1 1 1 -1 -1 -1 -1 1 1 1 1 1 -1 1 -1 1 1 -1 -1 1 1 -1 1 -1 1 1 1 -1 1 1 -1 -1 1 1 1 1 1 1 1 1 1 1 -1 -1 1 -1 -1 -1 1 1 -1 1 -1 -1 1 1 1 -1 -1 -1 1 -1 -1 -1 1 1 1 1 -1 -1 1 -1 1 1 1 -1 -1 -1 -1 -1 1 1 -1 1 -1 -1 -1 1 -1 -1 1 -1 -1 -1 -1 -1 1 1 -1 -1 -1 -1 -1 -1 1 -1 1 -1 1 -1 -1 1 -1 1 -1 -1 -1 -1 1 -1 -1 1 1 1 1 -1 1 1 1 -1 1 -1 1 1 -1 -1 -1 -1 1 1 1 -1 1 1 -1 -1 1 -1 -1 1 -1 -1 -1 -1 -1 1 -1 1 -1 -1 -1 -1 -1 -1]  InternalRulePriority=Speed  RndMeth=Simplest  InputSameDT=on
  PRN1 : Outport
  wires:
  Clock/1 -> Tabela de C/A/1
  Tabela de C/A/1 -> PRN1/1

== system satellite/Satelite 14 /Subsistema do código C//A/Satelites/Sat 12 ==
  Clock : Inport
  Action Port : ActionPort  ActionType=case
  Tabela de C/A : Lookup_n-D  NumberOfTableDimensions=1  BreakpointsForDimension1=[0,1,2,3,4,5,6,7,8,9,10,11,12,13,14,15,16,17,18,19,20,21,22,23,24,25,26,27,28,29,30,31,32,33,34,35,36,37,38,39,40,41,42,43,44,45,46,47,48,49,50,51,52,53,54,55,56,57,58,59,60,61,62,63,64,65,66,67,68,69,70,71,72,73,74,75,76,77,78,79,80,81,82,83,84,85,86,87,88,89,90,91,92,93,94,95,96,97,98,99,100,101,102,103,104,105,106,107,108,109,110,111,112,113,114,115,116,117,118,119,120,121,122,123,124,125,126,127,128,129,130,131,132,133,134,135,136,137,138,139,140,141,142,143,144,145,146,147,148,149,150,151,152,153,154,155,156,157,158,159,160,161,162,163,164,165,166,167,168,169,170,171,172,173,174,175,176,177,178,179,180,181,182,183,184,185,186,187,188,189,190,191,192,193,194,195,196,197,198,199,200,201,202,203,204,205,206,207,208,209,210,211,212,213,214,215,216,217,218,219,220,221,222,223,224,225,226,227,228,229,230,231,232,233,234,235,236,237,238,239,240,241,242,243,244,245,246,247,248,249,250,251,252,253,254,255,256,257,258,259,260,261,262,263,264,265,266,267,268,269,270,271,272,273,274,275,276,277,278,279,280,281,282,283,284,285,286,287,288,289,290,291,292,293,294,295,296,297,298,299,300,301,302,303,304,305,306,307,308,309,310,311,312,313,314,315,316,317,318,319,320,321,322,323,324,325,326,327,328,329,330,331,332,333,334,335,336,337,338,339,340,341,342,343,344,345,346,347,348,349,350,351,352,353,354,355,356,357,358,359,360,361,362,363,364,365,366,367,368,369,370,371,372,373,374,375,376,377,378,379,380,381,382,383,384,385,386,387,388,389,390,391,392,393,394,395,396,397,398,399,400,401,402,403,404,405,406,407,408,409,410,411,412,413,414,415,416,417,418,419,420,421,422,423,424,425,426,427,428,429,430,431,432,433,434,435,436,437,438,439,440,441,442,443,444,445,446,447,448,449,450,451,452,453,454,455,456,457,458,459,460,461,462,463,464,465,466,467,468,469,470,471,472,473,474,475,476,477,478,479,480,481,482,483,484,485,486,487,488,489,490,491,492,493,494,495,496,497,498,499,500,501,502,503,504,505,506,507,508,509,510,511,512,513,514,515,516,517,518,519,520,521,522,523,524,525,526,527,528,529,530,531,532,533,534,535,536,537,538,539,540,541,542,543,544,545,546,547,548,549,550,551,552,553,554,555,556,557,558,559,560,561,562,563,564,565,566,567,568,569,570,571,572,573,574,575,576,577,578,579,580,581,582,583,584,585,586,587,588,589,590,591,592,593,594,595,596,597,598,599,600,601,602,603,604,605,606,607,608,609,610,611,612,613,614,615,616,617,618,619,620,621,622,623,624,625,626,627,628,629,630,631,632,633,634,635,636,637,638,639,640,641,642,643,644,645,646,647,648,649,650,651,652,653,654,655,656,657,658,659,660,661,662,663,664,665,666,667,668,669,670,671,672,673,674,675,676,677,678,679,680,681,682,683,684,685,686,687,688,689,690,691,692,693,694,695,696,697,698,699,700,701,702,703,704,705,706,707,708,709,710,711,712,713,714,715,716,717,718,719,720,721,722,723,724,725,726,727,728,729,730,731,732,733,734,735,736,737,738,739,740,741,742,743,744,745,746,747,748,749,750,751,752,753,754,755,756,757,758,759,760,761,762,763,764,765,766,767,768,769,770,771,772,773,774,775,776,777,778,779,780,781,782,783,784,785,786,787,788,789,790,791,792,793,794,795,796,797,798,799,800,801,802,803,804,805,806,807,808,809,810,811,812,813,814,815,816,817,818,819,820,821,822,823,824,825,826,827,828,829,830,831,832,833,834,835,836,837,838,839,840,841,842,843,844,845,846,847,848,849,850,851,852,853,854,855,856,857,858,859,860,861,862,863,864,865,866,867,868,869,870,871,872,873,874,875,876,877,878,879,880,881,882,883,884,885,886,887,888,889,890,891,892,893,894,895,896,897,898,899,900,901,902,903,904,905,906,907,908,909,910,911,912,913,914,915,916,917,918,919,920,921,922,923,924,925,926,927,928,929,930,931,932,933,934,935,936,937,938,939,940,941,942,943,944,945,946,947,948,949,950,951,952,953,954,955,956,957,958,959,960,961,962,963,964,965,966,967,968,969,970,971,972,973,974,975,976,977,978,979,980,981,982,983,984,985,986,987,988,989,990,991,992,993,994,995,996,997,998,999,1000,1001,1002,1003,1004,1005,1006,1007,1008,1009,1010,1011,1012,1013,1014,1015,1016,1017,1018,1019,1020,1021,1022]  Table=[1,1,1,1,1,-1,1,-1,-1,-1,-1,1,1,-1,1,-1,1,1,1,-1,-1,-1,1,-1,-1,1,-1,-1,-1,-1,1,-1,-1,-1,1,1,1,1,-1,-1,-1,-1,1,-1,1,1,1,1,1,1,1,1,1,1,-1,1,1,1,1,1,-1,-1,1,-1,-1,1,-1,-1,1,1,1,1,-1,1,-1,-1,-1,-1,1,1,1,1,1,1,1,-1,1,1,-1,-1,-1,1,-1,1,1,-1,-1,-1,-1,-1,-1,-1,-1,1,1,-1,1,-1,-1,1,-1,1,1,1,1,-1,-1,1,1,-1,-1,-1,-1,-1,1,-1,1,-1,-1,1,1,1,1,-1,1,1,-1,-1,-1,-1,-1,1,-1,-1,-1,1,-1,1,1,1,-1,-1,-1,-1,1,-1,1,-1,-1,1,-1,-1,1,-1,1,-1,1,-1,1,-1,-1,1,1,-1,-1,1,1,-1,1,1,1,1,1,1,-1,1,1,-1,1,1,-1,1,1,1,1,-1,1,-1,-1,1,1,1,-1,-1,-1,1,1,-1,1,-1,-1,1,1,1,-1,1,1,1,-1,-1,-1,-1,1,1,-1,-1,1,-1,1,-1,-1,-1,1,1,1,-1,-1,1,-1,-1,-1,1,1,1,-1,-1,1,-1,1,-1,-1,-1,-1,1,1,-1,1,1,1,1,1,-1,-1,-1,1,-1,-1,1,1,-1,1,-1,-1,-1,1,-1,-1,1,1,1,1,-1,-1,1,1,1,1,-1,-1,1,-1,-1,-1,1,1,-1,1,1,1,1,-1,1,1,1,1,-1,-1,-1,1,1,-1,1,1,-1,-1,-1,1,-1,-1,1,1,1,1,-1,1,-1,1,-1,1,-1,1,-1,1,-1,1,-1,-1,-1,-1,1,1,-1,1,-1,1,1,-1,-1,-1,-1,-1,-1,1,1,-1,1,-1,1,-1,1,1,-1,-1,-1,-1,1,1,-1,-1,1,1,-1,1,-1,-1,-1,1,1,-1,1,1,-1,1,-1,1,1,1,1,-1,-1,1,1,1,-1,1,-1,-1,-1,1,-1,1,1,-1,-1,1,1,-1,1,1,-1,-1,1,1,-1,1,-1,-1,1,1,-1,1,-1,1,1,-1,-1,1,-1,-1,-1,-1,1,-1,-1,-1,1,-1,-1,1,1,-1,1,-1,-1,-1,1,-1,1,-1,-1,1,-1,1,-1,1,-1,1,-1,1,1,1,1,-1,1,1,1,1,-1,1,-1,-1,-1,1,1,-1,-1,1,1,1,-1,1,1,1,-1,1,-1,1,1,1,1,1,1,1,1,1,-1,1,-1,1,1,1,-1,-1,-1,-1,1,1,1,-1,-1,-1,1,1,-1,1,1,-1,1,-1,1,1,-1,1,-1,-1,-1,1,-1,-1,1,1,-1,1,-1,1,-1,1,1,1,-1,1,1,1,1,1,-1,1,1,1,-1,1,-1,1,-1,-1,1,1,-1,-1,-1,-1,1,-1,-1,-1,-1,-1,1,1,1,1,1,1,1,-1,1,1,-1,-1,1,-1,1,1,-1,1,-1,-1,1,-1,1,1,1,1,-1,-1,-1,-1,-1,-1,1,1,-1,-1,1,-1,-1,-1,-1,1,1,1,1,-1,-1,-1,-1,1,-1,-1,1,-1,-1,-1,1,1,-1,1,1,1,1,-1,-1,1,1,1,1,1,1,-1,1,-1,-1,1,1,1,-1,1,-1,-1,1,-1,-1,1,1,1,-1,1,1,-1,-1,-1,-1,-1,1,-1,1,1,1,1,1,-1,1,1,-1,-1,1,1,1,-1,-1,1,1,1,-1,1,-1,-1,-1,1,-1,-1,-1,-1,-1,-1,-1,-1,-1,-1,1,-1,1,-1,-1,1,-1,1,-1,-1,-1,1,1,1,1,-1,-1,1,-1,-1,1,1,1,-1,1,1,1,-1,-1,-1,1,1,-1,-1,-1,1,-1,-1,1,1,-1,1,-1,1,-1,1,1,1,1,1,1,1,1,-1,-1,-1,-1,-1,-1,1,1,1,-1,1,-1,-1,1,1,1,1,1,-1,-1,1,1,-1,1,-1,-1,-1,1,1,-1,1,-1,-1,1,-1,-1,-1,-1,-1,-1,-1,-1,1,-1,1,1,-1,-1,-1,1,1,-1,1,1,-1,1,1,1,-1,1,1,-1,-1,-1,1,-1,1,1,-1,1,1,-1,-1,1,-1,-1,1,-1,-1,-1,1,1,1,1,1,1,1,1,1,-1,-1,-1,1,-1,-1,1,-1,-1,1,-1,1,-1,1,1,1,1,-1,-1,-1,-1,1,-1,1,1,-1,-1,1,-1,-1,-1,-1,-1,1,-1,1,1,-1,1,-1,-1,-1,-1,1,1,-1,-1,-1,1,1,1,-1,-1,1,1,1,-1,1,1,-1,-1,1,-1,1,1,-1,-1,-1,1,-1,1,1,1,-1,1,-1,1,-1,1,1,-1,1,-1,1,-1,-1,-1,-1,-1,-1,1,1,1,-1,1,1,-1,1,1,-1,-1,1,-1,1,-1,1,-1,-1,-1,-1,1,-1,-1,-1,-1,1,1,-1,1,-1,1,1,-1,1,-1,1,-1,-1,1,1,1,-1,1,1,-1,-1,1,-1,1,-1,1,-1,-1,-1,-1,1,1,-1,-1,-1,1,-1,-1,-1,1,-1,1,-1,-1,-1,1,1,1,-1,-1,-1,1,-1,1,-1,-1,-1,1,1,-1,-1,1,1,-1,-1,-1,-1]  InternalRulePriority=Speed  RndMeth=Simplest  InputSameDT=on
  PRN12 : Outport
  wires:
  Clock/1 -> Tabela de C/A/1
  Tabela de C/A/1 -> PRN12/1

== system satellite/Satelite 14 /Subsistema do código C//A/Satelites/Sat 13 ==
  Clock : Inport
  Action Port : ActionPort  ActionType=case
  Tabela de C/A : Lookup_n-D  NumberOfTableDimensions=1  BreakpointsForDimension1=[0,1,2,3,4,5,6,7,8,9,10,11,12,13,14,15,16,17,18,19,20,21,22,23,24,25,26,27,28,29,30,31,32,33,34,35,36,37,38,39,40,41,42,43,44,45,46,47,48,49,50,51,52,53,54,55,56,57,58,59,60,61,62,63,64,65,66,67,68,69,70,71,72,73,74,75,76,77,78,79,80,81,82,83,84,85,86,87,88,89,90,91,92,93,94,95,96,97,98,99,100,101,102,103,104,105,106,107,108,109,110,111,112,113,114,115,116,117,118,119,120,121,122,123,124,125,126,127,128,129,130,131,132,133,134,135,136,137,138,139,140,141,142,143,144,145,146,147,148,149,150,151,152,153,154,155,156,157,158,159,160,161,162,163,164,165,166,167,168,169,170,171,172,173,174,175,176,177,178,179,180,181,182,183,184,185,186,187,188,189,190,191,192,193,194,195,196,197,198,199,200,201,202,203,204,205,206,207,208,209,210,211,212,213,214,215,216,217,218,219,220,221,222,223,224,225,226,227,228,229,230,231,232,233,234,235,236,237,238,239,240,241,242,243,244,245,246,247,248,249,250,251,252,253,254,255,256,257,258,259,260,261,262,263,264,265,266,267,268,269,270,271,272,273,274,275,276,277,278,279,280,281,282,283,284,285,286,287,288,289,290,291,292,293,294,295,296,297,298,299,300,301,302,303,304,305,306,307,308,309,310,311,312,313,314,315,316,317,318,319,320,321,322,323,324,325,326,327,328,329,330,331,332,333,334,335,336,337,338,339,340,341,342,343,344,345,346,347,348,349,350,351,352,353,354,355,356,357,358,359,360,361,362,363,364,365,366,367,368,369,370,371,372,373,374,375,376,377,378,379,380,381,382,383,384,385,386,387,388,389,390,391,392,393,394,395,396,397,398,399,400,401,402,403,404,405,406,407,408,409,410,411,412,413,414,415,416,417,418,419,420,421,422,423,424,425,426,427,428,429,430,431,432,433,434,435,436,437,438,439,440,441,442,443,444,445,446,447,448,449,450,451,452,453,454,455,456,457,458,459,460,461,462,463,464,465,466,467,468,469,470,471,472,473,474,475,476,477,478,479,480,481,482,483,484,485,486,487,488,489,490,491,492,493,494,495,496,497,498,499,500,501,502,503,504,505,506,507,508,509,510,511,512,513,514,515,516,517,518,519,520,521,522,523,524,525,526,527,528,529,530,531,532,533,534,535,536,537,538,539,540,541,542,543,544,545,546,547,548,549,550,551,552,553,554,555,556,557,558,559,560,561,562,563,564,565,566,567,568,569,570,571,572,573,574,575,576,577,578,579,580,581,582,583,584,585,586,587,588,589,590,591,592,593,594,595,596,597,598,599,600,601,602,603,604,605,606,607,608,609,610,611,612,613,614,615,616,617,618,619,620,621,622,623,624,625,626,627,628,629,630,631,632,633,634,635,636,637,638,639,640,641,642,643,644,645,646,647,648,649,650,651,652,653,654,655,656,657,658,659,660,661,662,663,664,665,666,667,668,669,670,671,672,673,674,675,676,677,678,679,680,681,682,683,684,685,686,687,688,689,690,691,692,693,694,695,696,697,698,699,700,701,702,703,704,705,706,707,708,709,710,711,712,713,714,715,716,717,718,719,720,721,722,723,724,725,726,727,728,729,730,731,732,733,734,735,736,737,738,739,740,741,742,743,744,745,746,747,748,749,750,751,752,753,754,755,756,757,758,759,760,761,762,763,764,765,766,767,768,769,770,771,772,773,774,775,776,777,778,779,780,781,782,783,784,785,786,787,788,789,790,791,792,793,794,795,796,797,798,799,800,801,802,803,804,805,806,807,808,809,810,811,812,813,814,815,816,817,818,819,820,821,822,823,824,825,826,827,828,829,830,831,832,833,834,835,836,837,838,839,840,841,842,843,844,845,846,847,848,849,850,851,852,853,854,855,856,857,858,859,860,861,862,863,864,865,866,867,868,869,870,871,872,873,874,875,876,877,878,879,880,881,882,883,884,885,886,887,888,889,890,891,892,893,894,895,896,897,898,899,900,901,902,903,904,905,906,907,908,909,910,911,912,913,914,915,916,917,918,919,920,921,922,923,924,925,926,927,928,929,930,931,932,933,934,935,936,937,938,939,940,941,942,943,944,945,946,947,948,949,950,951,952,953,954,955,956,957,958,959,960,961,962,963,964,965,966,967,968,969,970,971,972,973,974,975,976,977,978,979,980,981,982,983,984,985,986,987,988,989,990,991,992,993,994,995,996,997,998,999,1000,1001,1002,1003,1004,1005,1006,1007,1008,1009,1010,1011,1012,1013,1014,1015,1016,1017,1018,1019,1020,1021,1022]  Table=[1,1,1,1,1,1,-1,1,-1,-1,1,-1,1,-1,-1,1,1,1,1,-1,1,-1,1,1,-1,1,-1,-1,1,-1,1,-1,1,1,1,1,1,-1,-1,-1,-1,-1,1,-1,1,-1,-1,1,1,-1,1,1,1,-1,-1,1,1,-1,-1,-1,-1,1,1,1,-1,-1,1,1,1,-1,1,1,1,-1,1,-1,-1,1,1,-1,-1,-1,-1,-1,-1,-1,1,1,1,-1,1,1,-1,-1,1,1,1,-1,-1,1,1,1,-1,1,-1,1,-1,-1,-1,1,1,1,-1,-1,1,-1,1,1,-1,1,1,-1,1,-1,-1,1,1,-1,1,1,1,-1,1,1,1,1,-1,-1,1,-1,-1,-1,1,-1,1,-1,-1,1,-1,-1,-1,1,1,1,-1,-1,-1,-1,-1,1,1,1,-1,-1,1,-1,1,1,1,1,-1,-1,1,-1,1,1,1,-1,-1,1,-1,1,1,1,-1,1,1,1,1,1,-1,1,1,-1,1,-1,1,1,-1,1,-1,-1,-1,-1,1,-1,-1,-1,-1,1,-1,1,-1,1,1,1,-1,-1,-1,1,1,-1,-1,-1,1,1,-1,-1,-1,-1,-1,-1,1,-1,1,1,1,1,1,-1,1,-1,-1,1,1,1,1,-1,1,-1,-1,1,-1,-1,-1,-1,1,1,1,1,1,-1,-1,-1,-1,-1,1,-1,-1,-1,-1,1,1,-1,-1,1,1,-1,-1,1,1,-1,1,-1,-1,-1,-1,-1,-1,1,-1,1,-1,1,1,-1,-1,-1,-1,-1,1,-1,-1,-1,1,1,1,1,1,1,-1,1,-1,1,1,1,1,1,-1,1,-1,-1,1,-1,-1,-1,-1,1,1,-1,1,1,1,1,-1,1,-1,-1,1,1,-1,-1,-1,-1,1,1,-1,1,1,-1,-1,-1,-1,-1,-1,-1,1,-1,-1,-1,1,-1,-1,1,-1,-1,-1,1,1,1,1,1,1,-1,-1,1,-1,1,1,1,1,1,-1,-1,-1,-1,-1,1,-1,-1,-1,-1,1,-1,1,-1,-1,1,-1,1,1,-1,1,-1,-1,-1,1,1,-1,1,-1,-1,1,1,-1,-1,-1,1,1,1,1,1,-1,-1,1,1,1,-1,1,1,-1,1,-1,1,1,-1,1,-1,1,-1,1,-1,1,1,1,-1,-1,1,-1,-1,1,-1,-1,1,-1,1,1,-1,1,-1,1,1,-1,-1,1,-1,-1,-1,-1,1,1,-1,1,-1,1,-1,-1,-1,1,1,-1,1,-1,-1,-1,-1,1,-1,-1,-1,-1,-1,1,1,-1,-1,1,1,-1,1,-1,-1,-1,1,-1,1,1,1,-1,-1,1,-1,1,1,-1,-1,1,-1,1,-1,-1,1,-1,-1,-1,1,1,1,1,1,-1,-1,1,1,1,1,1,-1,-1,1,-1,1,-1,1,-1,-1,1,1,1,-1,-1,1,-1,1,1,1,-1,-1,1,-1,1,1,1,1,-1,1,-1,1,1,1,1,-1,1,-1,-1,1,-1,1,1,1,1,-1,-1,-1,1,1,-1,1,-1,1,-1,-1,1,1,-1,-1,-1,1,1,1,1,1,1,-1,1,1,-1,1,-1,-1,-1,1,1,1,-1,1,1,-1,1,-1,1,1,-1,1,-1,-1,-1,1,1,1,1,1,-1,-1,1,-1,-1,1,-1,1,1,-1,1,-1,1,1,-1,1,1,1,1,1,-1,-1,-1,1,1,-1,-1,-1,1,-1,-1,-1,-1,-1,-1,1,-1,-1,-1,1,-1,-1,-1,1,1,1,1,1,1,-1,1,1,1,-1,-1,1,1,-1,-1,-1,1,-1,1,-1,-1,-1,1,1,1,1,1,-1,-1,1,-1,1,1,1,-1,1,-1,1,1,1,-1,1,-1,1,1,1,1,-1,1,-1,1,-1,1,1,1,-1,1,-1,1,1,-1,1,-1,-1,1,1,-1,-1,1,1,-1,1,-1,1,-1,-1,1,-1,-1,-1,1,-1,1,-1,-1,1,1,-1,-1,1,1,1,1,-1,-1,-1,-1,1,1,1,1,-1,1,1,-1,-1,1,-1,1,-1,-1,1,1,-1,-1,-1,1,1,1,-1,-1,1,1,-1,-1,-1,-1,-1,1,1,-1,1,1,-1,-1,-1,1,1,1,-1,1,1,-1,1,-1,-1,1,-1,1,-1,1,1,-1,1,-1,-1,-1,-1,-1,1,-1,1,1,-1,1,1,1,1,1,-1,-1,1,-1,1,1,-1,-1,1,-1,-1,1,-1,1,1,-1,1,1,1,1,1,1,-1,-1,-1,-1,1,-1,-1,-1,1,-1,1,1,1,1,1,1,-1,1,-1,1,1,1,1,-1,1,1,1,1,-1,-1,1,-1,1,-1,-1,-1,1,1,-1,-1,1,1,1,1,1,-1,1,1,-1,-1,1,-1,-1,-1,1,1,-1,-1,-1,-1,1,-1,-1,-1,-1,-1,-1,1,-1,-1,-1,-1,-1,-1,-1,-1,1,-1,1,1,-1,-1,-1,-1,-1,1,-1,-1,-1,1,-1,1,1,-1,-1,-1,-1,-1,-1,-1,-1,1,1,1,-1,1,1,-1,-1,1,-1,1,-1,1,1,1,1,-1,1,-1,1,-1,-1,-1,-1,1,1,-1,1,-1,-1,1,1,-1,-1,-1,-1,1,-1,-1,-1,1,1,1,-1,-1,1,1,1,1,-1,1,1,-1,-1,-1]  InternalRulePriority=Speed  RndMeth=Simplest  InputSameDT=on
  PRN13 : Outport
  wires:
  Clock/1 -> Tabela de C/A/1
  Tabela de C/A/1 -> PRN13/1
